simulink model "simulasyon"  (R2017a)
settings: Solver=ode4  StartTime=0.0  StopTime=0.05  FixedStep=1e-8  MaxStep=1e-4  RelTol=1e-3
libraries: powerlib x16, powerlib_meascontrol x3
settings Model: Creator=Hakan Polat  LastModifiedBy=user

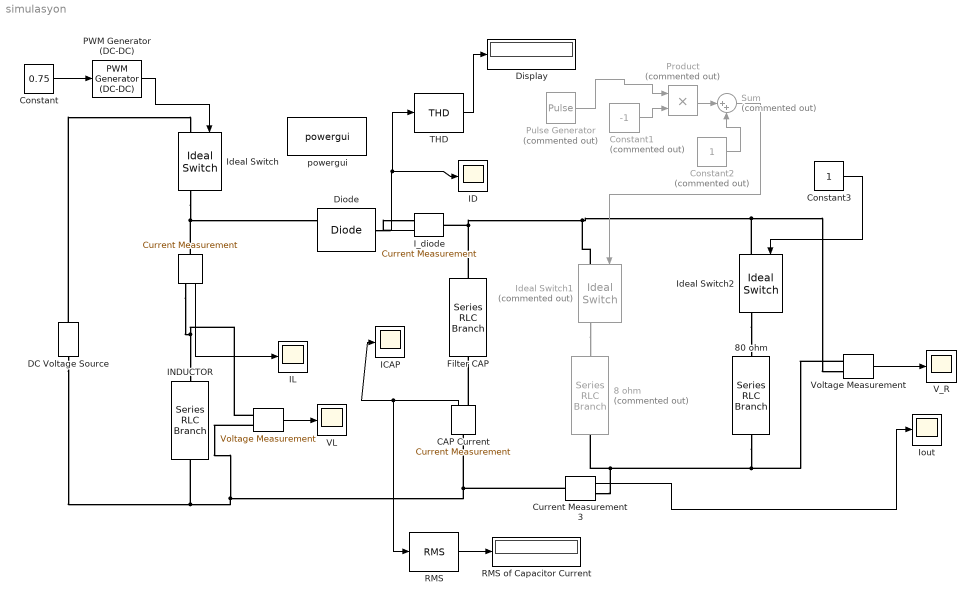
== system simulasyon ==
  " " : powerlib/Measurements/Voltage Measurement  PhasorSimulation=off  OutputType=Complex  PSBequivalent=0
  " " : powerlib/Measurements/Current Measurement  PhasorSimulation=off  OutputType=Complex  PSBequivalent=0
  "8 ohm " : powerlib/Elements/Series RLC Branch  Commented=on  LConnTagsString=__new0  RConnTagsString=__new0  BranchType=R  Resistance=8  Inductance=1e-3  SetiL0=off  InitialCurrent=0  Capacitance=1e-6  Setx0=off  InitialVoltage=0  Measurements=None
  80 ohm : powerlib/Elements/Series RLC Branch  LConnTagsString=__new0  RConnTagsString=__new0  BranchType=R  Resistance=80  Inductance=1e-3  SetiL0=off  InitialCurrent=0  Capacitance=1e-6  Setx0=off  InitialVoltage=0  Measurements=None
  "CAP Current " : powerlib/Measurements/Current Measurement  PhasorSimulation=off  OutputType=Complex  PSBequivalent=0
  Constant : Constant  Value=0.75
  Constant1 : Constant  Commented=on  Value=-1
  Constant2 : Constant  Commented=on
  Constant3 : Constant
  Current Measurement3 : powerlib/Measurements/Current Measurement  PhasorSimulation=off  OutputType=Complex  PSBequivalent=0
  DC Voltage Source : powerlib/Electrical Sources/DC Voltage Source  Amplitude=8.5  Measurements=None
  Diode : powerlib/Power Electronics/Diode  Ron=0.001  Lon=0  Vf=0.8  IC=0  UseSnubber=0  Rs=500  Cs=250e-9  Measurements=on
  Display : Display
  Filter CAP : powerlib/Elements/Series RLC Branch  LConnTagsString=__new0  RConnTagsString=__new0  BranchType=C  Resistance=1  Inductance=1e-3  SetiL0=off  InitialCurrent=0  Capacitance=100e-6  Setx0=off  InitialVoltage=0  Measurements=None
  ICAP : Scope
  ID : Scope
  IL : Scope
  INDUCTOR : powerlib/Elements/Series RLC Branch  LConnTagsString=__new0  RConnTagsString=__new0  BranchType=RL  Resistance=10e-3  Inductance=10e-6  SetiL0=off  InitialCurrent=0  Capacitance=1e-6  Setx0=off  InitialVoltage=0  Measurements=None
  I_diode : powerlib/Measurements/Current Measurement  PhasorSimulation=off  OutputType=Complex  PSBequivalent=0
  Ideal Switch : powerlib/Power Electronics/Ideal Switch  Ron=0.001  Lon=0  IC=0  Rs=1e5  Cs=inf  Measurements=on
  Ideal Switch1 : powerlib/Power Electronics/Ideal Switch  Commented=on  Ron=0.001  Lon=0  IC=0  Rs=1e5  Cs=inf  Measurements=on
  Ideal Switch2 : powerlib/Power Electronics/Ideal Switch  Ron=0.001  Lon=0  IC=0  Rs=1e5  Cs=inf  Measurements=on
  Iout : Scope
  PWM Generator (DC-DC) : powerlib_meascontrol/Pulse & Signal Generators/PWM Generator (DC-DC)  Fsw=100000  Ts=0
  Product : Product  Commented=on
  Pulse Generator : DiscretePulseGenerator  Commented=on  PulseType=Time based  Period=10  PulseWidth=5  PhaseDelay=10e-3
  RMS : powerlib_meascontrol/Measurements/RMS  TrueRMS=on  Freq=100000  RMSInit=120  Ts=0
  RMS of Capacitor Current : Display
  Sum : Sum  Commented=on  Inputs=|++
  THD : powerlib_meascontrol/Measurements/THD  Freq=100000  Ts=0
  VL : Scope
  V_R : Scope
  Voltage Measurement : powerlib/Measurements/Voltage Measurement  PhasorSimulation=off  OutputType=Complex  PSBequivalent=0
  powergui : powerlib/powergui  Priority=1  SimulationMode=Discrete  SampleTime=1e-8  frequency=60  Iterations=50  frequencyindice=0  Pbase=100e6  ErrMax=1e-4  UnitsV=kV  UnitsW=MW  buscounter=0  FunctionMessages=off  echomessages=off  EnableUseOfTLC=off  CurrentSourceSwitches=off  DisableSnubberDevices=off  DisableRonSwitches=off  DisableVfSwitches=off  DisplayEquations=off  SolverType=Tustin/Backward Euler (TBE)  Interpol=off  ExternalGateDelay=off  methode=off  Ts=100  x0status=blocks  SPID=on  SwTol=0  HookPort=off  RestoreLinks=warning  ResistiveCurrentMeasurement=off  Frange=[0:2:500]  Ylog=off  Xlog=on  ShowGrid=off  save=off  variable=ZData  structure=I_capa  ZoomFFT=on  StartTime=0.02  cycles=200  DisplayStyle=1  fundamental=100000  FreqAxis=on  MaxFrequency=2000000  frequencyindicesteady=1  RmsSteady=1  display=off
  wires:
  Constant/1 -> PWM Generator (DC-DC)/1
  Voltage Measurement/1 -> V_R/1
  " "/1 -> VL/1
  " "/1 -> IL/1
  Current Measurement3/1 -> Iout/1
  "CAP Current "/1 -> RMS/1, ICAP/1
  THD/1 -> Display/1
  Constant1/1 -> Product/2
  Product/1 -> Sum/1
  Constant2/1 -> Sum/2
  I_diode/1 -> ID/1, THD/1
  PWM Generator (DC-DC)/1 -> Ideal Switch/1
  RMS/1 -> RMS of Capacitor Current/1
  Sum/1 -> Ideal Switch1/1
  Pulse Generator/1 -> Product/1
  Constant3/1 -> Ideal Switch2/1
  connections:
  Ideal Switch/RConn1 -- " "/LConn1 -- Diode/RConn1
  DC Voltage Source/RConn1 -- Ideal Switch/LConn1
  Voltage Measurement/LConn1 -- 80 ohm/RConn1 -- Current Measurement3/RConn1 -- "8 ohm "/RConn1
  Filter CAP/RConn1 -- I_diode/LConn1 -- Ideal Switch1/LConn1 -- Ideal Switch2/LConn1 -- Voltage Measurement/LConn2
  Diode/LConn1 -- I_diode/RConn1
  " "/LConn1 -- " "/RConn1 -- INDUCTOR/LConn1
  "CAP Current "/RConn1 -- Filter CAP/LConn1
  INDUCTOR/RConn1 -- DC Voltage Source/LConn1 -- " "/LConn2 -- Current Measurement3/LConn1 -- "CAP Current "/LConn1
  Ideal Switch1/RConn1 -- "8 ohm "/LConn1
  Ideal Switch2/RConn1 -- 80 ohm/LConn1
